simulink model "CoolingCheese_5thPoint"  (R2022a)
settings: Solver=VariableStepAuto  StartTime=0.0  StopTime=H  RelTol=1e-3
undefined symbols (not defined in the file): C_c, C_f, k_af, k_fc, q_MAX, q_min, theta0_c, theta0_f, Ts, var_wc, var_wf
libraries: slpidlib x1
settings Model: Creator=mrnel  LastModifiedBy=mrnel

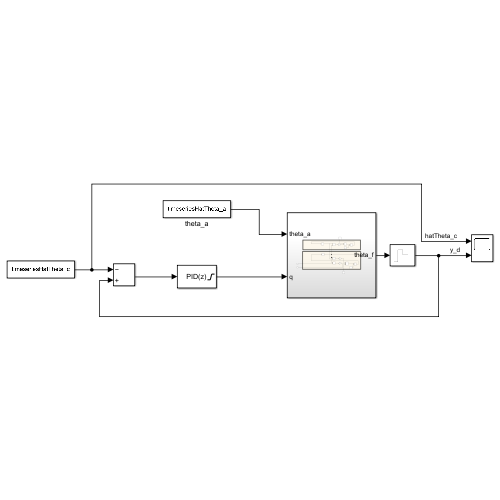
[thumbnail: Simulink's stored preview of the top-level diagram]
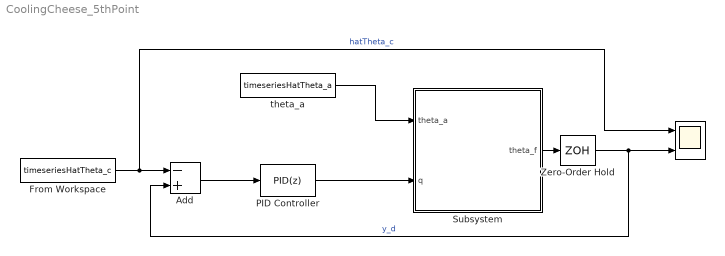
== system CoolingCheese_5thPoint ==
  " " : Scope  NumInputPorts=2
  Add : Sum  Inputs=-+
  From Workspace : FromWorkspace  VariableName=timeseriesHatTheta_c  SampleTime=Ts
  PID Controller : slpidlib/PID Controller  Controller=PID  Form=Parallel  TimeDomain=Discrete-time  UseExternalTs=off  SampleTime=Ts  IntegratorMethod=Forward Euler  FilterMethod=Forward Euler  ControllerParametersSource=internal  P=-9.49221780957707  I=-0.011735630152087  UseKiTs=off  D=864.504912629527  N=0.0109132825594137  UseFilter=on  TunerSelectOption=Transfer Function Based (PID Tuner App)  InitialConditionSource=internal  InitialConditionForIntegrator=0  InitialConditionForFilter=0  DifferentiatorICPrevScaledInput=0  ExternalReset=none  TrackingMode=off  Kt=1  LimitOutput=on  SatLimitsSource=internal  UpperSaturationLimit=q_MAX  LowerSaturationLimit=q_min  LinearizeAsGain=on  AntiWindupMode=none  Kb=1  POutMin=[]  POutMax=[]  IOutMin=[]  IOutMax=[]  DOutMin=[]  DOutMax=[]  NOutMin=[]  NOutMax=[]  SumOutMin=[]  SumOutMax=[]  SaturationOutMin=[]  SaturationOutMax=[]  PParamMin=[]  PParamMax=[]  IParamMin=[]  IParamMax=[]  DParamMin=[]  DParamMax=[]  NParamMin=[]  NParamMax=[]  KbParamMin=[]  KbParamMax=[]  KtParamMin=[]  KtParamMax=[]  KbOutMin=[]  KbOutMax=[]  KtOutMin=[]  KtOutMax=[]  IntegratorOutMin=[]  IntegratorOutMax=[]  FilterOutMin=[]  FilterOutMax=[]  SumI1OutMin=[]  SumI1OutMax=[]  SumI2OutMin=[]  SumI2OutMax=[]  SumI3OutMin=[]  SumI3OutMax=[]  SumI4OutMin=[]  SumI4OutMax=[]  SumDOutMin=[]  SumDOutMax=[]  DifferentiatorOutMin=[]  DifferentiatorOutMax=[]  FilterDiffOutCoefMin=[]  FilterDiffOutCoefMax=[]  ReciprocalOutMin=[]  ReciprocalOutMax=[]  SumDenOutMin=[]  SumDenOutMax=[]  SumNumOutMin=[]  SumNumOutMax=[]  DivideOutMin=[]  DivideOutMax=[]  UdiffTsProdOutMin=[]  UdiffTsProdOutMax=[]  NTsProdOutMin=[]  NTsProdOutMax=[]  UintegralTsProdOutMin=[]  UintegralTsProdOutMax=[]  UngainTsProdOutMin=[]  UngainTsProdOutMax=[]  IntegratorContinuousStateAttributes=''  IntegratorStateMustResolveToSignalObject=off  IntegratorRTWStateStorageClass=Auto  FilterContinuousStateAttributes=''  FilterStateMustResolveToSignalObject=off  FilterRTWStateStorageClass=Auto  ParallelPVariant=InternalParameters  IdealPVariant=Disabled  IVariant=InternalParameters  DVariant=InternalParameters  IntegratorVariant=Discrete  SatVariant=Enabled  AWVariant=Passthrough  PCopyVariant=Disabled  TRVariant=Disabled  FdbkBlocksVariant=Forward  IdealPFdbkVariant=Disabled  SatFdbkVariant=Disabled  DerivativeFilterVariant=ForwardEulerFilter  NVariant=InternalParameters  NCopyVariant=Disabled  FilterICVariant=InternalICsFilter  IntegratorICVariant=InternalICs  ExternalResetVariant=Disabled  TRSumVariant=Passthrough  SumFdbkVariant=Disabled  SumVariant=Sum_PID  TsampFilterVariant=InternalTs  TsampNgainVariant=Passthrough  TsampIntegralVariant=Passthrough  ExternalSaturationOutDataTypeStr=Inherit: Same as second input  aMode=0
  Subsystem : Subsystem
  Zero-Order Hold : ZeroOrderHold  SampleTime=Ts
  theta_a : FromWorkspace  VariableName=timeseriesHatTheta_a  SampleTime=Ts
  wires:
  theta_a/1 -> Subsystem/1(theta_a)
  PID Controller/1 -> Subsystem/2(q)
  Subsystem/1(theta_f) -> Zero-Order Hold/1
  Zero-Order Hold/1 -> Add/2, " "/2  "y_d"
  From Workspace/1 -> " "/1, Add/1  "hatTheta_c"
  Add/1 -> PID Controller/1

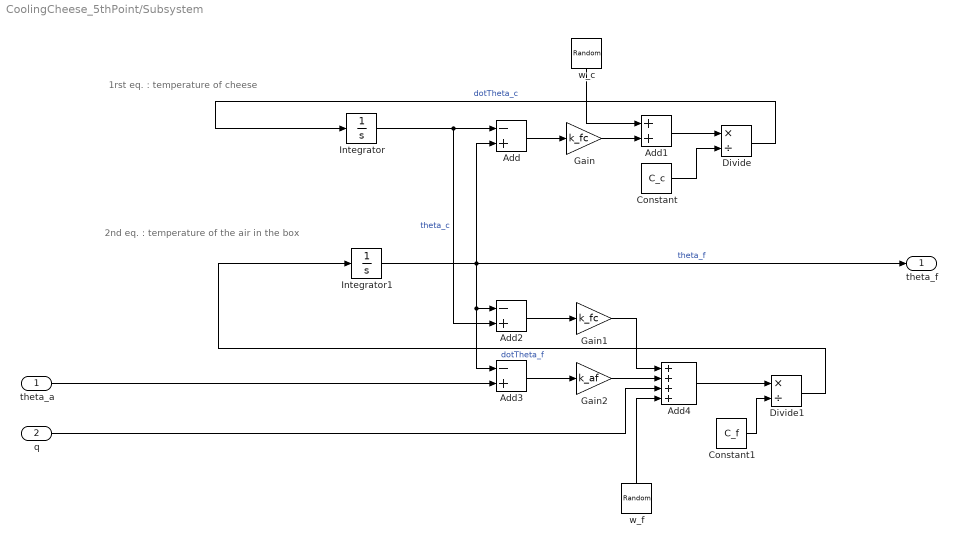
== system CoolingCheese_5thPoint/Subsystem ==
  note: 2nd eq. : temperature of the air in the box
  note: 1rst eq. : temperature of cheese
  theta_a : Inport
  q : Inport  Port=2
  Add : Sum  Inputs=-+
  Add1 : Sum
  Add2 : Sum  Inputs=-+
  Add3 : Sum  Inputs=-+
  Add4 : Sum  Inputs=++++
  Constant : Constant  Value=C_c
  Constant1 : Constant  Value=C_f
  Divide : Product  Inputs=*/
  Divide1 : Product  Inputs=*/
  Gain : Gain  Gain=k_fc
  Gain1 : Gain  Gain=k_fc
  Gain2 : Gain  Gain=k_af
  Integrator : Integrator  InitialCondition=theta0_c
  Integrator1 : Integrator  InitialCondition=theta0_f
  w_c : RandomNumber  Variance=var_wc  SampleTime=Ts
  w_f : RandomNumber  Variance=var_wf  SampleTime=Ts
  theta_f : Outport
  wires:
  Gain2/1 -> Add4/2
  Divide/1 -> Integrator/1  "dotTheta_c"
  Add2/1 -> Gain1/1
  Add1/1 -> Divide/1
  Divide1/1 -> Integrator1/1  "dotTheta_f"
  w_c/1 -> Add1/1
  Integrator/1 -> Add2/2, Add/1  "theta_c"
  Integrator1/1 -> theta_f/1, Add3/1, Add2/1, Add/2  "theta_f"
  Gain/1 -> Add1/2
  Add/1 -> Gain/1
  Constant1/1 -> Divide1/2
  w_f/1 -> Add4/4
  Constant/1 -> Divide/2
  Gain1/1 -> Add4/1
  Add3/1 -> Gain2/1
  Add4/1 -> Divide1/1
  q/1 -> Add4/3
  theta_a/1 -> Add3/2
